simulink model "punto_e2"  (R2014a)
settings: Solver=ode45  StartTime=0.0  StopTime=50.0  RelTol=1e-3
values from neighbouring files (symbols this model uses):
  Kc = 1    [es1.m]
  Kr = 1    [es1.m]
libraries: simulink x2, cstblocks x1
settings Model: Creator=HP  LastModifiedBy=HP

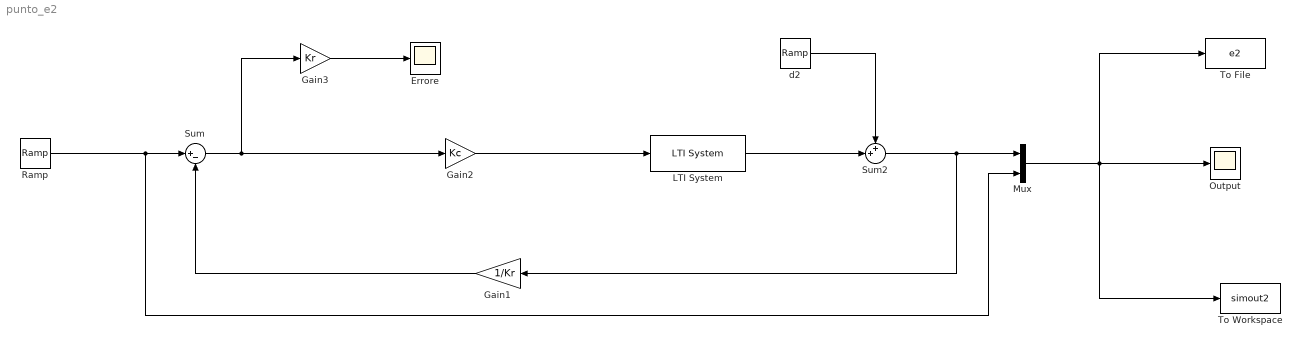
== system punto_e2 ==
  Errore : Scope
  Gain1 : Gain  Gain=1/Kr
  Gain2 : Gain  Gain=Kc
  Gain3 : Gain  Gain=Kr
  LTI System : cstblocks/LTI System  sys=F  IC=[]
  Mux : Mux  Inputs=2
  Output : Scope
  Ramp : simulink/Sources/Ramp  slope=2  start=0  X0=0
  Sum : Sum  Inputs=|+-
  Sum2 : Sum  Inputs=++|
  To File : ToFile  Filename=e2  MatrixName=output  SaveFormat=Timeseries
  To Workspace : ToWorkspace  VariableName=simout2  SaveFormat=Timeseries  SampleTime=-1
  d2 : simulink/Sources/Ramp  slope=0.01  start=0  X0=0
  wires:
  Sum/1 -> Gain3/1, Gain2/1
  Gain1/1 -> Sum/2
  LTI System/1 -> Sum2/2
  Sum2/1 -> Gain1/1, Mux/1
  Mux/1 -> To File/1, To Workspace/1, Output/1
  Ramp/1 -> Mux/2, Sum/1
  Gain3/1 -> Errore/1
  Gain2/1 -> LTI System/1
  d2/1 -> Sum2/1
